simulink model "obsreducido"  (R2020b)
settings: Solver=VariableStepAuto  StartTime=0.0  StopTime=5  RelTol=1e-3
undefined symbols (not defined in the file): National_Instruments, PCI
libraries: sldrtlib x2, simulink x1
settings Model: Creator=diosdado  LastModifiedBy=diosdado
settings SolverCC: ZeroCrossAlgorithm=Adaptive
settings DebuggingCC: IgnoredZcDiagnostic=none

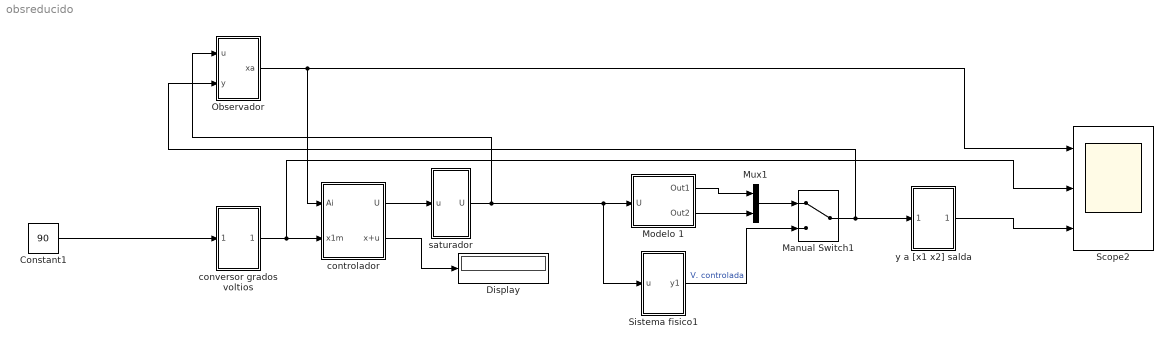
== system obsreducido ==
  Constant1 : Constant  Value=90
  Display : Display
  Manual Switch1 : ManualSwitch
  Modelo 1 : Subsystem
  Mux1 : Mux  Inputs=2
  Observador : Subsystem
  Scope2 : Scope  NumInputPorts=3
  Sistema fisico1 : Subsystem
  controlador : Subsystem
  "conversor grados voltios " : Subsystem  mask{a=1, b=0}
  saturador : Subsystem
  y a [x1 x2] salda : Subsystem  mask{a=4.92, b=0.82}
  wires:
  Modelo 1/2(Out2) -> Mux1/2
  controlador/2(x+u) -> Display/1
  controlador/1(U) -> saturador/1(u)
  Sistema fisico1/1(y1) -> Manual Switch1/2  "V. controlada"
  saturador/1(U) -> Observador/1(u), Sistema fisico1/1(u), Modelo 1/1(U)
  Modelo 1/1(Out1) -> Mux1/1
  Mux1/1 -> Manual Switch1/1
  Manual Switch1/1 -> Observador/2(y), y a [x1 x2] salda/1(In1)
  "conversor grados voltios "/1(Out1) -> Scope2/2, controlador/2(x1m)
  Constant1/1 -> "conversor grados voltios "/1(In1)
  Observador/1(xa) -> Scope2/1, controlador/1(Ai)
  y a [x1 x2] salda/1(Out1) -> Scope2/3

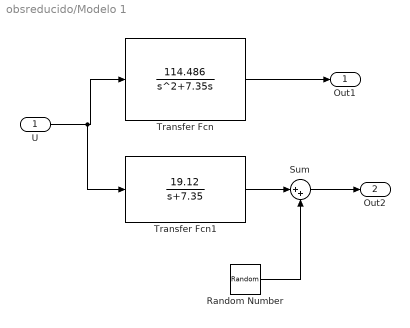
== system obsreducido/Modelo 1 ==
  U : Inport
  Random Number : RandomNumber  Variance=0.01  SampleTime=0.01
  Sum : Sum  Inputs=|++
  Transfer Fcn : TransferFcn  Numerator=[114.486]  Denominator=[1 7.35 0]
  Transfer Fcn1 : TransferFcn  Numerator=[19.12]  Denominator=[1 7.35]
  Out1 : Outport
  Out2 : Outport  Port=2
  wires:
  U/1 -> Transfer Fcn1/1, Transfer Fcn/1
  Transfer Fcn/1 -> Out1/1
  Transfer Fcn1/1 -> Sum/1
  Random Number/1 -> Sum/2
  Sum/1 -> Out2/1

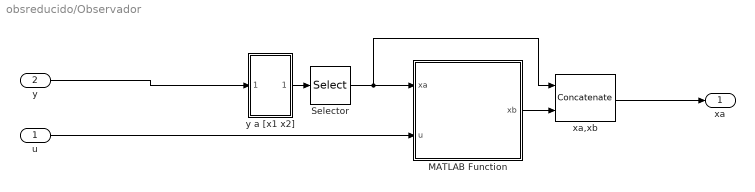
== system obsreducido/Observador ==
  u : Inport
  y : Inport  Port=2
  MATLAB Function : MATLAB Function  TreatAsAtomicUnit=on
  Selector : Selector  InputPortWidth=2  IndexOptions=Index vector (dialog)  Indices=[1]  OutputSizes=1
  xa,xb : Concatenate  ConcatenateDimension=2
  y a [x1 x2] : Subsystem  mask{a=4.92, b=0.82}
  xa : Outport
  wires:
  Selector/1 -> xa,xb/1, MATLAB Function/1(xa)
  u/1 -> MATLAB Function/2(u)
  MATLAB Function/1(xb) -> xa,xb/2
  y a [x1 x2]/1(Out1) -> Selector/1
  xa,xb/1 -> xa/1
  y/1 -> y a [x1 x2]/1(In1)

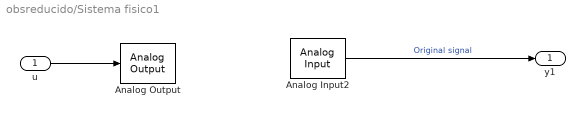
== system obsreducido/Sistema fisico1 ==
  u : Inport
  Analog Input2 : sldrtlib/Analog Input  SampleTime=0.001  MaxMissedTicks=10  ShowMissedTicks=off  YieldWhenWaiting=off  DrvName=National_Instruments/PCI-6014  DrvAddress=4294967295  DrvOptions=[2 0 0 0 0 0]  Channels=[1,2]  RangeMode=1  VoltRange=1  DataType=1
      settings: AttributesFormatString=National Instruments\nPCI-6014 [auto]
  Analog Output : sldrtlib/Analog Output  SampleTime=0.001  MaxMissedTicks=10  ShowMissedTicks=off  YieldWhenWaiting=off  DrvName=National_Instruments/PCI-6014  DrvAddress=4294967295  DrvOptions=[2 0 0 0 0 0]  Channels=1  RangeMode=1  VoltRange=1  InitialValue=[]  FinalValue=[]
      settings: AttributesFormatString=National Instruments\nPCI-6014 [auto]
  y1 : Outport
  wires:
  u/1 -> Analog Output/1
  Analog Input2/1 -> y1/1  "Original signal"

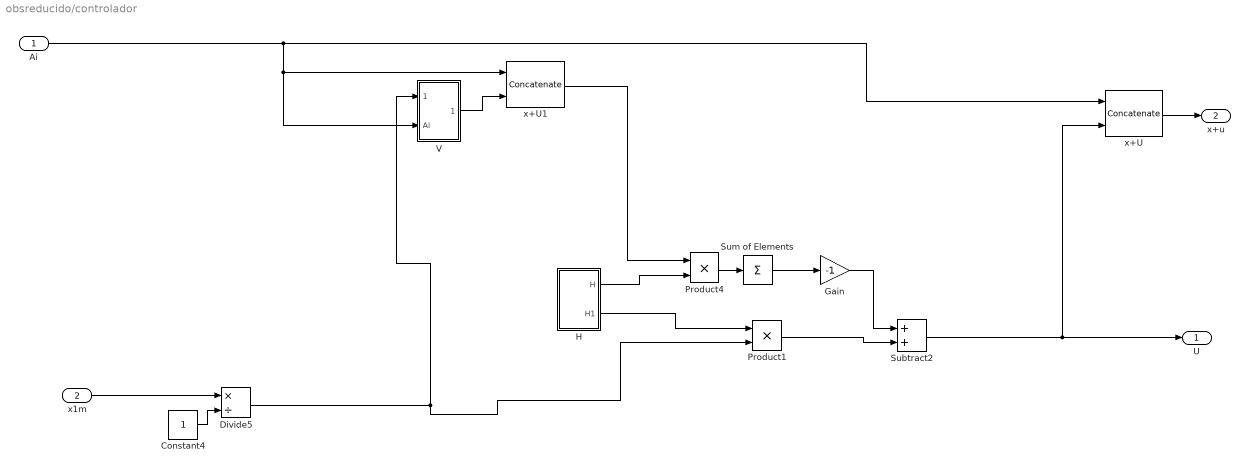
== system obsreducido/controlador ==
  Ai : Inport  OutDataTypeStr=double
  x1m : Inport  Port=2
  Constant4 : Constant
  Divide5 : Product  Inputs=*/
  Gain : Gain  Gain=-1
  H : Subsystem  mask{h1=15.349, h2=0.769, h3=-0.019}
  Product1 : Product
  Product4 : Product
  Subtract2 : Sum  OutDataTypeStr=double
  Sum of Elements : Sum  Inputs=+
  V : Subsystem
  x+U : Concatenate  ConcatenateDimension=2
  x+U1 : Concatenate  ConcatenateDimension=2
  U : Outport  OutDataTypeStr=double
  x+u : Outport  Port=2
  wires:
  Product4/1 -> Sum of Elements/1
  Gain/1 -> Subtract2/1
  Divide5/1 -> Product1/2, V/1(In2)
  H/1(H) -> Product4/2
  H/2(H1) -> Product1/1
  Sum of Elements/1 -> Gain/1
  Product1/1 -> Subtract2/2
  x+U/1 -> x+u/1
  V/1(Out1) -> x+U1/2
  x+U1/1 -> Product4/1
  Ai/1 -> x+U/1, V/2(Ai), x+U1/1
  Constant4/1 -> Divide5/2
  x1m/1 -> Divide5/1
  Subtract2/1 -> x+U/2, U/1

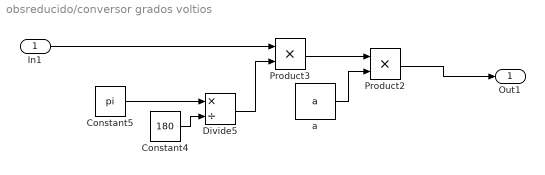
== system obsreducido/conversor grados voltios  ==
  In1 : Inport
  Constant4 : Constant  Value=180
  Constant5 : Constant  Value=pi
  Divide5 : Product  Inputs=*/
  Product2 : Product
  Product3 : Product
  a : Constant  Value=a
  Out1 : Outport
  wires:
  Product3/1 -> Product2/1
  Constant4/1 -> Divide5/2
  In1/1 -> Product3/1
  a/1 -> Product2/2
  Constant5/1 -> Divide5/1
  Divide5/1 -> Product3/2
  Product2/1 -> Out1/1

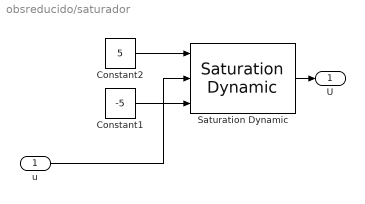
== system obsreducido/saturador ==
  u : Inport  OutDataTypeStr=double
  Constant1 : Constant  Value=-5
  Constant2 : Constant  Value=5
  Saturation Dynamic : simulink/Discontinuities/Saturation Dynamic  OutMin=-5  OutMax=5  OutDataTypeStr=Inherit: Same as second input  OutDataType=fixdt(1, 16)  OutScaling=2^-10  DoSatur=off
  U : Outport  OutDataTypeStr=double
  wires:
  u/1 -> Saturation Dynamic/2
  Constant2/1 -> Saturation Dynamic/1
  Saturation Dynamic/1 -> U/1
  Constant1/1 -> Saturation Dynamic/3

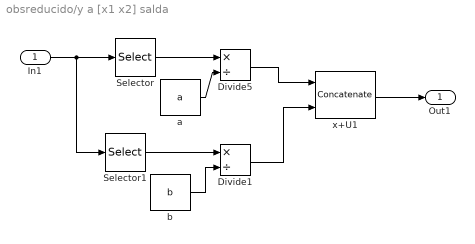
== system obsreducido/y a [x1 x2] salda ==
  In1 : Inport
  Divide1 : Product  Inputs=*/
  Divide5 : Product  Inputs=*/
  Selector : Selector  InputPortWidth=2  IndexOptions=Index vector (dialog)  Indices=[1]  OutputSizes=1
  Selector1 : Selector  InputPortWidth=2  IndexOptions=Index vector (dialog)  Indices=[2]  OutputSizes=1
  a : Constant  Value=a
  b : Constant  Value=b
  x+U1 : Concatenate  ConcatenateDimension=2
  Out1 : Outport
  wires:
  In1/1 -> Selector1/1, Selector/1
  a/1 -> Divide5/2
  Selector/1 -> Divide5/1
  Selector1/1 -> Divide1/1
  b/1 -> Divide1/2
  Divide5/1 -> x+U1/1
  Divide1/1 -> x+U1/2
  x+U1/1 -> Out1/1

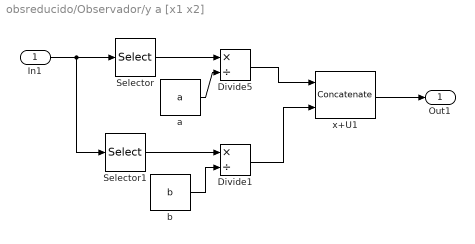
== system obsreducido/Observador/y a [x1 x2] ==
  In1 : Inport
  Divide1 : Product  Inputs=*/
  Divide5 : Product  Inputs=*/
  Selector : Selector  InputPortWidth=2  IndexOptions=Index vector (dialog)  Indices=[1]  OutputSizes=1
  Selector1 : Selector  InputPortWidth=2  IndexOptions=Index vector (dialog)  Indices=[2]  OutputSizes=1
  a : Constant  Value=a
  b : Constant  Value=b
  x+U1 : Concatenate  ConcatenateDimension=2
  Out1 : Outport
  wires:
  In1/1 -> Selector1/1, Selector/1
  a/1 -> Divide5/2
  Selector/1 -> Divide5/1
  Selector1/1 -> Divide1/1
  b/1 -> Divide1/2
  Divide5/1 -> x+U1/1
  Divide1/1 -> x+U1/2
  x+U1/1 -> Out1/1

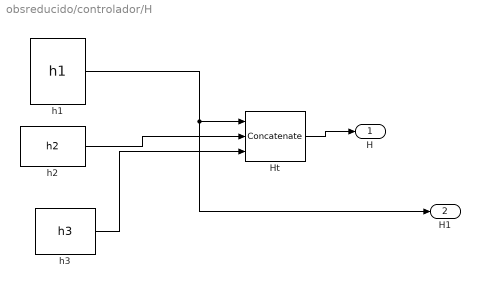
== system obsreducido/controlador/H ==
  Ht : Concatenate  NumInputs=3  ConcatenateDimension=2
  h1 : Constant  Value=h1
  h2 : Constant  Value=h2
  h3 : Constant  Value=h3
  H : Outport
  H1 : Outport  Port=2
  wires:
  h1/1 -> H1/1, Ht/1
  h2/1 -> Ht/2
  Ht/1 -> H/1
  h3/1 -> Ht/3

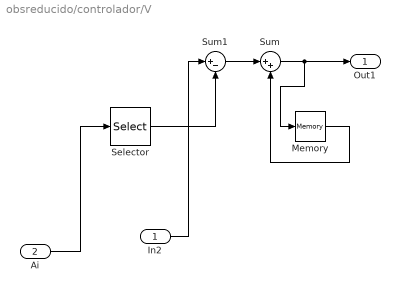
== system obsreducido/controlador/V ==
  In2 : Inport
  Ai : Inport  Port=2  PortDimensions=2
  Memory : Memory  InheritSampleTime=on  LinearizeAsDelay=on
  Selector : Selector  InputPortWidth=2  IndexOptions=Index vector (dialog)  Indices=[1]  OutputSizes=1
  Sum : Sum  Inputs=|++
  Sum1 : Sum  Inputs=|+-
  Out1 : Outport
  wires:
  In2/1 -> Sum1/1
  Sum/1 -> Out1/1, Memory/1
  Sum1/1 -> Sum/1
  Memory/1 -> Sum/2
  Ai/1 -> Selector/1
  Selector/1 -> Sum1/2

== matlab function obsreducido/Observador/MATLAB Function ==
  data: xa input; xb output; u input
function xb = fcn(xa,u)
L=39.713;
Abb=-7.35;
Aab=1;
Aaa=0;
Aba=0;
Bb=23.317;
Ba=0;
  n=(1/( Abb-L*Aab))*((Bb-L*Ba)*u+(Aba+L*Aaa+Abb*L-L*Aab*L)*xa);
 xb=n+L*xa;
end
